simulink library "ESTS_BRK"  (R2024b)
settings: Solver=VariableStepAuto  StartTime=0.0  StopTime=10.0  RelTol=1e-3
undefined symbols (not defined in the file or in its folder): ESTS_BRK_p_TqBrkLoLim_Nm, ESTS_BRK_p_TqBrkUpLim_Nm, p_BrkTqGainFr_Nmpbar, p_BrkTqGainRe_Nmpbar
libraries: simulink x1
settings Model: Creator=blatak  LastModifiedBy=blatak

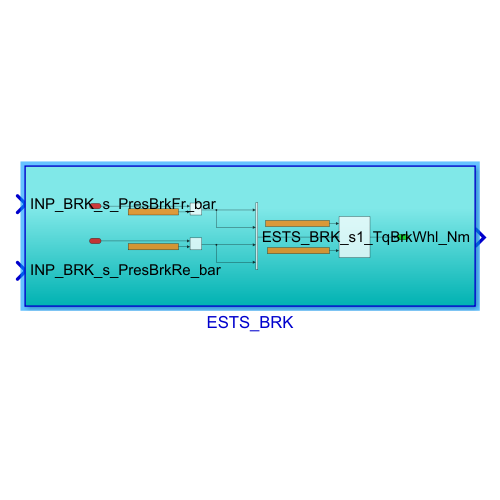
[thumbnail: Simulink's stored preview of the top-level diagram]
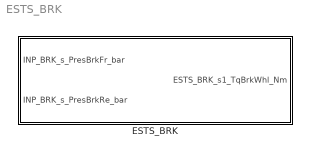
== system ESTS_BRK ==
  ESTS_BRK : Subsystem

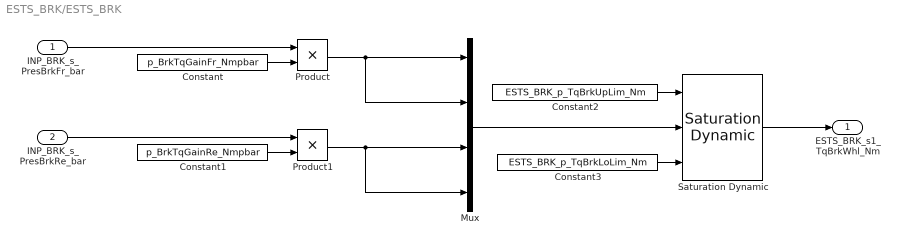
== system ESTS_BRK/ESTS_BRK ==
  INP_BRK_s_PresBrkFr_bar : Inport
  INP_BRK_s_PresBrkRe_bar : Inport  Port=2
  Constant : Constant  Value=p_BrkTqGainFr_Nmpbar
  Constant1 : Constant  Value=p_BrkTqGainRe_Nmpbar
  Constant2 : Constant  Value=ESTS_BRK_p_TqBrkUpLim_Nm
  Constant3 : Constant  Value=ESTS_BRK_p_TqBrkLoLim_Nm
  Mux : Mux
  Product : Product
  Product1 : Product
  Saturation Dynamic : simulink/Discontinuities/Saturation Dynamic  OutMin=[]  OutMax=[]  OutDataTypeStr=Inherit: Same as second input  OutDataType=fixdt(1, 16)  OutScaling=2^-10  DoSatur=off
  ESTS_BRK_s1_TqBrkWhl_Nm : Outport
  wires:
  Product/1 -> Mux/2, Mux/1
  Constant/1 -> Product/2
  INP_BRK_s_PresBrkFr_bar/1 -> Product/1
  Product1/1 -> Mux/4, Mux/3
  Constant1/1 -> Product1/2
  INP_BRK_s_PresBrkRe_bar/1 -> Product1/1
  Mux/1 -> Saturation Dynamic/2
  Saturation Dynamic/1 -> ESTS_BRK_s1_TqBrkWhl_Nm/1
  Constant2/1 -> Saturation Dynamic/1
  Constant3/1 -> Saturation Dynamic/3
